simulink model "gm_encoderN8withDelay"  (R2016b)
settings: Solver=FixedStepDiscrete  StartTime=0.0  StopTime=10.0  RelTol=1e-3
settings Model: Creator=hasee  LastModifiedBy=hasee
settings DataIOCC: LimitDataPoints=on  SaveOutput=off  SaveTime=off
settings OptimizationCC: BlockReduction=off  ConditionallyExecuteInputs=off  DefaultParameterBehavior=Inlined  LifeSpan=inf
settings DebuggingCC: AlgebraicLoopMsg=error  InheritedTsInSrcMsg=none  SingleTaskRateTransMsg=error  AllowSymbolicDim=off  StrictBusMsg=ErrorOnBusTreatedAsVector  SFUnexpectedBacktrackingDiag=warning  SFNoUnconditionalDefaultTransitionDiag=warning  SFExecutionAtInitializationDiag=none
settings HardwareCC: ProdBitPerPointer=32  ProdBitPerSizeT=32  ProdBitPerPtrDiffT=32  ProdLargestAtomicFloat=None  ProdIntDivRoundTo=Undefined  ProdEndianess=Unspecified  ProdWordSize=32  ProdHWDeviceType=ASIC/FPGA->ASIC/FPGA  ProdEqTarget=off
settings GRTTargetCC: TargetLangStandard=C89/C90 (ANSI)  GeneratePreprocessorConditionals=Disable all
settings ConfigComp: CovScope=ReferencedModels  CovMetricSettings=dw  CovHtmlReporting=on  CovSaveCumulativeToWorkspaceVar=on  CovSaveSingleToWorkspaceVar=on  CovExternalEMLEnable=off  CovSFcnEnable=off

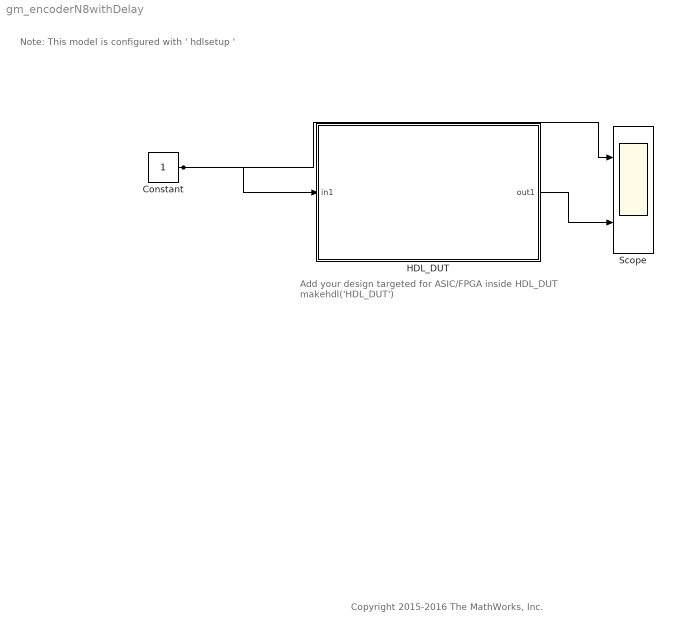
== system gm_encoderN8withDelay ==
  note: Copyright 2015-2016 The MathWorks, Inc.
  note: Add your design targeted for ASIC/FPGA inside HDL_DUT
      | makehdl('HDL_DUT')
  note: Note: This model is configured with ' hdlsetup '
  Constant : Constant  OutDataTypeStr=int8  SampleTime=-1
  HDL_DUT : Subsystem
  Scope : Scope  NumInputPorts=2
  wires:
  HDL_DUT/1(out1) -> Scope/2
  Constant/1 -> HDL_DUT/1(in1), Scope/1

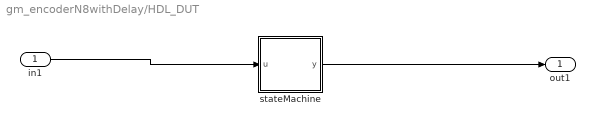
== system gm_encoderN8withDelay/HDL_DUT ==
  in1 : Inport
  stateMachine : Stateflow chart  TreatAsAtomicUnit=on
  out1 : Outport
  wires:
  in1/1 -> stateMachine/1(u)
  stateMachine/1(y) -> out1/1

== stateflow chart gm_encoderN8withDelay/HDL_DUT/stateMachine ==
  settings: executeAtInitialization=1
  state state1
    entry: y=true;
  state state2
    entry: y=false;
  (default) -> state1
  state2 -> state1 : [u<2]
  state1 -> state2 : [u>2]
  data: u input; y output boolean
